simulink model "V.1.3.SystemsmModelling_Modified_Aircorn"  (R2020a)
settings: Solver=ode23t  StartTime=0.0  StopTime=2000  MaxStep=2000.0  RelTol=1e-3
values from neighbouring files (symbols this model uses):
  InitialTemp = 300    [Setup.m]
undefined symbols (not defined in the file or in its folder): commanded_mass_flow, compressor_time_constant, condenser_length, copper_density, environment_temperature, evaporator_length, ground_temperature, pipe_diameter, pipe_thickness, target_temperature, temperature_delta, u_sat
libraries: fl_lib x55, nesl_utility x8, refrigeration_lib x1
(part 1 of 3)
settings Model: Creator=denni  LastModifiedBy=denni

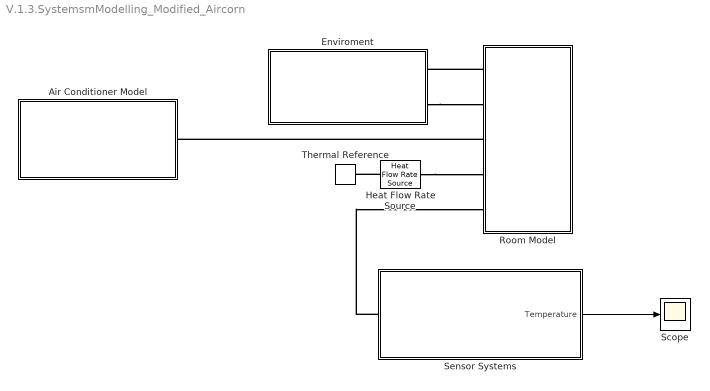
== system V.1.3.SystemsmModelling_Modified_Aircorn ==
  Air Conditioner Model : Subsystem
  Enviroment : Subsystem
  Heat Flow Rate Source : fl_lib/Thermal/Thermal Sources/Heat Flow Rate Source  heat_flow=10 W
      settings: SourceProductBaseCode=SS  InternalSimscapePortConfiguration="{\"Bottom\":[],\"Left\":[{\"id\":\"B\",\"label\":\"B\",\"type\":\"foundation.thermal.thermal\"}],\"Right\":[{\"id\":\"A\",\"label\":\"A\",\"type\":\"foundation.thermal.thermal\"}],\"Top\":[]}"
  Room Model : Subsystem
  Scope : Scope
  Sensor Systems : Subsystem
  Thermal Reference : fl_lib/Thermal/Thermal Elements/Thermal Reference
  wires:
  Sensor Systems/1("Temperature ") -> Scope/1
  connections:
  Room Model/LConn1 -- Enviroment/LConn1
  Enviroment/LConn2 -- Room Model/LConn2
  Room Model/LConn3 -- Air Conditioner Model/LConn1
  Sensor Systems/LConn1 -- Room Model/LConn5
  Heat Flow Rate Source/LConn1 -- Room Model/LConn4
  Heat Flow Rate Source/RConn1 -- Thermal Reference/LConn1
